simulink model "pre_lab3_2017b_"  (R2017b)
settings: Solver=VariableStepAuto  StartTime=0.0  StopTime=10.0  RelTol=1e-3
values from neighbouring files (symbols this model uses):
  atraso = stt    [manoel_outubro2.m]    (also in naao_roda.m = infor.SettlingTime; pre6_teste.m = infor.SettlingTime; pre_lab3.m = infor.SettlingTime; pre_lab3_lab.m = infor.SettlingTime)
  b0 = 18    [naao_roda.m]    (also in pre6_teste.m; pre_lab3.m; pre_lab3_2.m; pre_lab3_lab.m)
  ganho = 0.01027*infor.SettlingMax    [manoel_outubro2.m]    (also in naao_roda.m; pre6_teste.m; pre_lab3.m; pre_lab3_lab.m)
  Kpf = 1.0436    [pre_lab3.m]    (also in pre_lab3_lab.m; pre_lab4.m; pre_pedro.m = 1/dcgain(EE))
  q0c = 0.4    [naao_roda.m]
  q1 = q0*a1    [pre_lab3_2.m]    (also in pre_lab4.m; pre_lab4_2.m)
  R0 = round(r0,1)    [naao_roda.m]    (also in pre6_teste.m; pre_lab3.m; pre_lab3_lab.m; pre_lab4.m)
  T0 = round(t0,3)    [naao_roda.m]    (also in pre6_teste.m = 0.063; pre_lab3.m; pre_lab3_2.m = 0.0640576; pre_lab3_lab.m)
  Umax = 10    [naao_roda.m]    (also in pre6_teste.m; pre_lab3.m; pre_lab3_lab.m; pre_lab4.m)
settings Model: Creator=joaovitor  LastModifiedBy=joaovitor

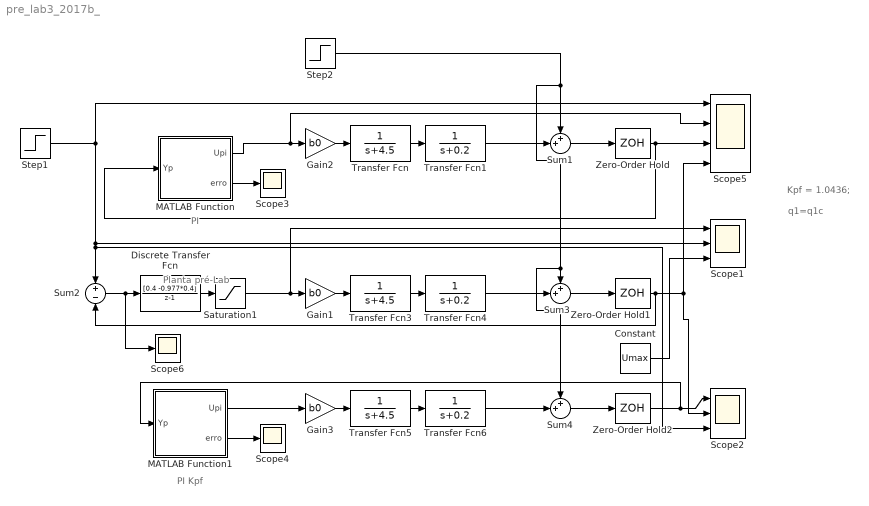
== system pre_lab3_2017b_ ==
  note: q1=q1c
  note: Kpf = 1.0436;
  note: Planta pré-Lab
  note: PI
  note: PI Kpf
  Constant : Constant  Value=Umax
  Discrete Transfer Fcn : DiscreteTransferFcn  Numerator=[0.4 -0.977*0.4]  Denominator=[1 -1]  SampleTime=T0
  Gain1 : Gain  Gain=b0
  Gain2 : Gain  Gain=b0
  Gain3 : Gain  Gain=b0
  MATLAB Function : MATLAB Function  TreatAsAtomicUnit=on
  MATLAB Function1 : MATLAB Function  TreatAsAtomicUnit=on
  Saturation1 : Saturate  UpperLimit=10  LowerLimit=-10
  Scope1 : Scope  NumInputPorts=3
  Scope2 : Scope  NumInputPorts=3
  Scope3 : Scope
  Scope4 : Scope
  Scope5 : Scope  NumInputPorts=4
  Scope6 : Scope
  Step1 : Step  Time=0  After=R0  SampleTime=0
  Step2 : Step  Time=2*3*atraso  After=10*ganho  SampleTime=0
  Sum1 : Sum  Inputs=++|
  Sum2 : Sum  Inputs=+|-
  Sum3 : Sum  Inputs=++|
  Sum4 : Sum  Inputs=++|
  Transfer Fcn : TransferFcn  Denominator=[1 4.5]
  Transfer Fcn1 : TransferFcn  Denominator=[1 0.2]
  Transfer Fcn3 : TransferFcn  Denominator=[1 4.5]
  Transfer Fcn4 : TransferFcn  Denominator=[1 0.2]
  Transfer Fcn5 : TransferFcn  Denominator=[1 4.5]
  Transfer Fcn6 : TransferFcn  Denominator=[1 0.2]
  Zero-Order Hold : ZeroOrderHold  SampleTime=T0
  Zero-Order Hold1 : ZeroOrderHold  SampleTime=T0
  Zero-Order Hold2 : ZeroOrderHold  SampleTime=T0
  wires:
  MATLAB Function/1(Upi) -> Scope5/2, Gain2/1
  Gain2/1 -> Transfer Fcn/1
  Transfer Fcn/1 -> Transfer Fcn1/1
  Transfer Fcn1/1 -> Sum1/2
  Sum1/1 -> Zero-Order Hold/1
  Step2/1 -> Sum4/1, Sum3/1, Sum1/1
  Step1/1 -> Scope5/1, Sum2/1, Scope2/3, Scope1/2
  Zero-Order Hold/1 -> MATLAB Function/1(Yp), Scope5/3
  MATLAB Function/2(erro) -> Scope3/1
  Discrete Transfer Fcn/1 -> Saturation1/1
  Transfer Fcn3/1 -> Transfer Fcn4/1
  Gain1/1 -> Transfer Fcn3/1
  Saturation1/1 -> Scope1/1, Gain1/1
  Transfer Fcn4/1 -> Sum3/2
  Sum3/1 -> Zero-Order Hold1/1
  Zero-Order Hold1/1 -> Sum2/2, Scope2/2, Scope5/4
  Transfer Fcn5/1 -> Transfer Fcn6/1
  Gain3/1 -> Transfer Fcn5/1
  Transfer Fcn6/1 -> Sum4/2
  Sum4/1 -> Zero-Order Hold2/1
  Zero-Order Hold2/1 -> MATLAB Function1/1(Yp), Scope2/1
  Constant/1 -> Scope1/3
  MATLAB Function1/1(Upi) -> Gain3/1
  MATLAB Function1/2(erro) -> Scope4/1
  Sum2/1 -> Scope6/1, Discrete Transfer Fcn/1

== matlab function pre_lab3_2017b_/MATLAB Function1 ==
  data: Upi output; Yp input; erro output; R0 parameter; q0c parameter; q1 parameter; Umax parameter; Kpf parameter
function [Upi,erro] = fcn(Yp, R0, q0c, q1, Umax, Kpf)    
persistent u0 e0 

if isempty(u0)
    u0=0;
    e0=0;
end

erro=1.1*Kpf*R0-Yp
Upi=u0+q0c*erro-q1*q0c*e0;

if(abs(Upi)>Umax)
    Upi=Umax*sign(Upi)

u0=Upi;
e0=erro;

end

== matlab function pre_lab3_2017b_/MATLAB Function ==
  data: Yp input; Upi output; erro output; R0 parameter; q0c parameter; Umax parameter; Kpf parameter; q1 parameter
function [Upi,erro] = fcn(Yp, R0, q0c, Umax, Kpf, q1)    
  
persistent u0; 
persistent e0;

if isempty(u0)
    u0=0;
    e0=0;
end

erro=R0-Yp
Upi=u0+q0c*erro-q1*q0c*e0;

if(abs(Upi)>Umax)
    Upi=Umax*sign(Upi)

u0=Upi;
e0=erro;

end
